simulink model "Ejercicio1Boolean"  (R2024b)
settings: Solver=VariableStepAuto  StartTime=0.0  StopTime=10.0  RelTol=1e-3
settings Model: Creator=user  LastModifiedBy=user

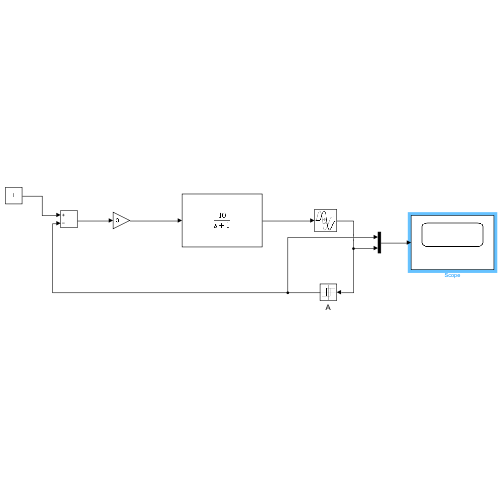
[thumbnail: Simulink's stored preview of the top-level diagram]
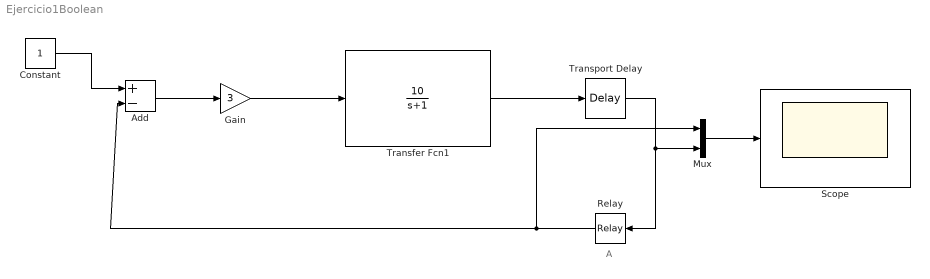
== system Ejercicio1Boolean ==
  note: A
  Add : Sum  Inputs=+-
  Constant : Constant
  Gain : Gain  Gain=3
  Mux : Mux  Inputs=2
  Relay : Relay  OnSwitchValue=5  OffSwitchValue=5
  Scope : Scope
  Transfer Fcn1 : TransferFcn  Numerator=[10]  Denominator=[1 1]
  Transport Delay : TransportDelay  DelayTime=0.01
  wires:
  Gain/1 -> Transfer Fcn1/1
  Transfer Fcn1/1 -> Transport Delay/1
  Constant/1 -> Add/1
  Relay/1 -> Mux/1, Add/2
  Add/1 -> Gain/1
  Transport Delay/1 -> Mux/2, Relay/1
  Mux/1 -> Scope/1
